simulink model "ex1"  (R2023b)
settings: Solver=VariableStepAuto  StartTime=0.0  StopTime=10.0  RelTol=1e-3
settings SolverCC: AlgebraicLoopSolver=TrustRegion
settings DebuggingCC: UnconnectedInputMsg=warning  UnconnectedOutputMsg=warning  UnconnectedLineMsg=warning
settings ModelReferenceCC: EnableRefExpFcnMdlSchedulingChecks=on

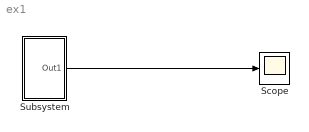
== system ex1 ==
  Scope : Scope
  Subsystem : Subsystem  mask{a=8}
      mask prompts: a "a="
      mask Callback a:
      | if str2num(get_param(gcb,'a'))<8
      |     error('Eroare');
      | end
      | 
      | if str2num(get_param(gcb,'a'))>10
      |     error('Eroare');
      | end
  wires:
  Subsystem/1(Out1) -> Scope/1

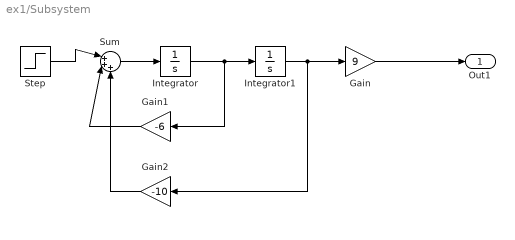
== system ex1/Subsystem ==
  Gain : Gain  Gain=9  ParamMin=[8]  ParamMax=[10]
  Gain1 : Gain  Gain=-6
  Gain2 : Gain  Gain=-10
  Integrator : Integrator
  Integrator1 : Integrator
  Step : Step  SampleTime=0
  Sum : Sum  Inputs=|+++
  Out1 : Outport
  wires:
  Gain1/1 -> Sum/2
  Integrator/1 -> Gain1/1, Integrator1/1
  Sum/1 -> Integrator/1
  Gain2/1 -> Sum/3
  Integrator1/1 -> Gain2/1, Gain/1
  Step/1 -> Sum/1
  Gain/1 -> Out1/1
